simulink model "model_testslx_2022a"  (R2022a)
settings: Solver=FixedStepAuto  StartTime=0.0  StopTime=100.0  FixedStep=0.01  RelTol=1e-3
undefined symbols (not defined in the file): beta, g, I, K, tau, U
settings Model: Creator=turgo  LastModifiedBy=micha

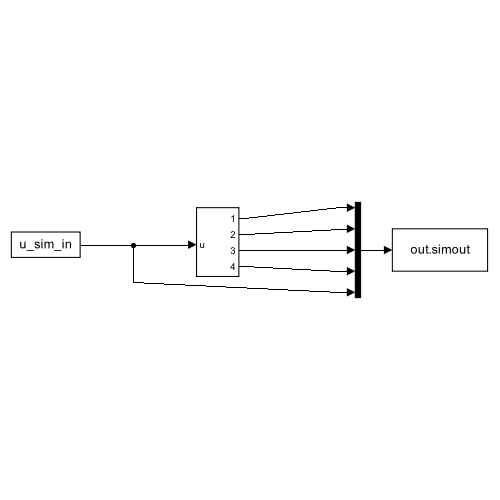
[thumbnail: Simulink's stored preview of the top-level diagram]
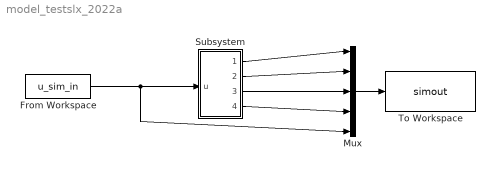
== system model_testslx_2022a ==
  From Workspace : FromWorkspace  VariableName=u_sim_in
  Mux : Mux  Inputs=5
  Subsystem : Subsystem
  To Workspace : ToWorkspace  VariableName=simout  SaveFormat=Structure With Time  SampleTime=-1
  wires:
  Mux/1 -> To Workspace/1
  Subsystem/1(Out1) -> Mux/1
  Subsystem/2(Out2) -> Mux/2
  Subsystem/3(Out3) -> Mux/3
  Subsystem/4(Out4) -> Mux/4
  From Workspace/1 -> Mux/5, Subsystem/1(u)

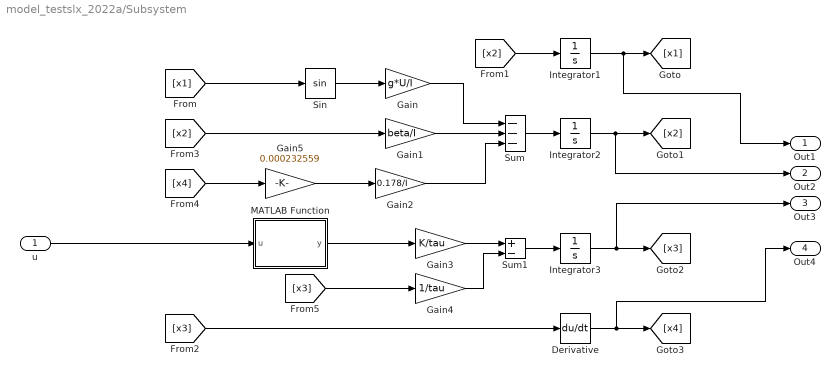
== system model_testslx_2022a/Subsystem ==
  u : Inport
  Derivative : Derivative
  Gain : Gain  Gain=g*U/I
  Gain1 : Gain  Gain=beta/I
  Gain2 : Gain  Gain=0.178/I
  Gain3 : Gain  Gain=K/tau
  Gain4 : Gain  Gain=1/tau
  Gain5 : Gain  Gain=0.000232559
  Integrator1 : Integrator
  Integrator2 : Integrator
  Integrator3 : Integrator
  MATLAB Function : MATLAB Function  TreatAsAtomicUnit=on
  Sin : Trigonometry
  Sum : Sum  Inputs=---
  Sum1 : Sum  Inputs=+-
  Out1 : Outport
  Out2 : Outport  Port=2
  Out3 : Outport  Port=3
  Out4 : Outport  Port=4
  wires:
  [x1] -> Sin/1
  Integrator1/1 -> Out1/1, [x1]
  Sum/1 -> Integrator2/1
  Sum1/1 -> Integrator3/1
  Sin/1 -> Gain/1
  Gain/1 -> Sum/1
  Gain2/1 -> Sum/3
  Gain4/1 -> Sum1/2
  Gain3/1 -> Sum1/1
  [x2] -> Gain1/1
  [x2] -> Integrator1/1
  Integrator3/1 -> Out3/1, [x3]
  Gain1/1 -> Sum/2
  Integrator2/1 -> Out2/1, [x2]
  u/1 -> MATLAB Function/1(u)
  Gain5/1 -> Gain2/1
  [x4] -> Gain5/1
  MATLAB Function/1(y) -> Gain3/1
  Derivative/1 -> Out4/1, [x4]
  [x3] -> Derivative/1
  [x3] -> Gain4/1

== matlab function model_testslx_2022a/Subsystem/MATLAB Function ==
  data: u input; y output
function y = fcn(u)

y = 211.6*u + 0.953;
